simulink model "simpleprocess_controller_observer"  (Simulink 7.4)
settings: Solver=ode45  StartTime=0.0  StopTime=10.0  RelTol=1e-3
values from neighbouring files (symbols this model uses):
  Kr1 = K_ret(2)    [auslegung.m]
  Kr2 = K_ret(3)    [auslegung.m]
  Kr3 = K_ret(1)    [auslegung.m]
  Kv = 24    [auslegung.m]
undefined symbols (not defined in the file or in its folder): Kb1, Kb2, Kb3, MU1
settings Model: Creator=Alex  LastModifiedBy=Alex

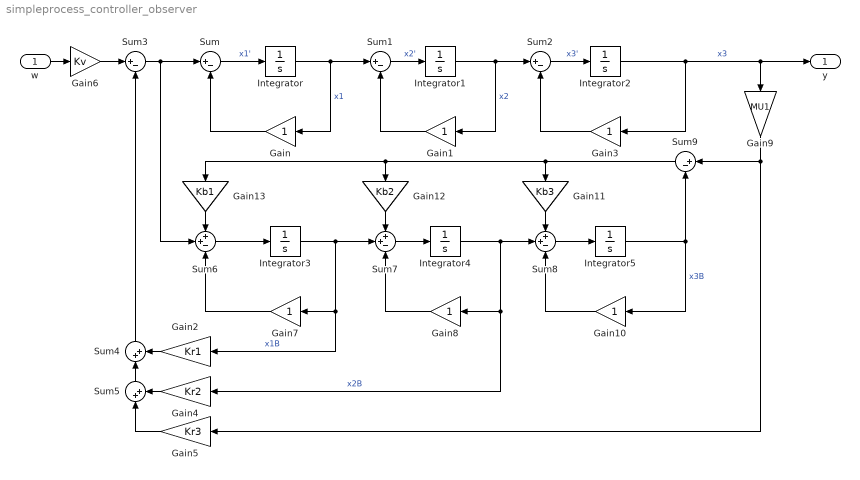
== system simpleprocess_controller_observer ==
  w : Inport  OutDataType=fixdt(1, 16)  OutScaling=2^0
  Gain{,1,3,7..8,10} (6 alike) : Gain  ParameterDataType=fixdt(1, 16)  ParameterScaling=2^0  OutDataType=fixdt(1, 16)  OutScaling=2^0
  Gain11 : Gain  Gain=Kb3  ParameterDataType=fixdt(1, 16)  ParameterScaling=2^0  OutDataType=fixdt(1, 16)  OutScaling=2^0
  Gain12 : Gain  Gain=Kb2  ParameterDataType=fixdt(1, 16)  ParameterScaling=2^0  OutDataType=fixdt(1, 16)  OutScaling=2^0
  Gain13 : Gain  Gain=Kb1  ParameterDataType=fixdt(1, 16)  ParameterScaling=2^0  OutDataType=fixdt(1, 16)  OutScaling=2^0
  Gain2 : Gain  Gain=Kr1  ParameterDataType=fixdt(1, 16)  ParameterScaling=2^0  OutDataType=fixdt(1, 16)  OutScaling=2^0
  Gain4 : Gain  Gain=Kr2  ParameterDataType=fixdt(1, 16)  ParameterScaling=2^0  OutDataType=fixdt(1, 16)  OutScaling=2^0
  Gain5 : Gain  Gain=Kr3  ParameterDataType=fixdt(1, 16)  ParameterScaling=2^0  OutDataType=fixdt(1, 16)  OutScaling=2^0
  Gain6 : Gain  Gain=Kv  ParameterDataType=fixdt(1, 16)  ParameterScaling=2^0  OutDataType=fixdt(1, 16)  OutScaling=2^0
  Gain9 : Gain  Gain=MU1  ParameterDataType=fixdt(1, 16)  ParameterScaling=2^0  OutDataType=fixdt(1, 16)  OutScaling=2^0
  Integrator{,1..5} (6 alike) : Integrator
  Sum{,1..3,9} (5 alike) : Sum  Inputs=|+-  OutDataType=fixdt(1, 16)  OutScaling=2^0
  Sum4 : Sum  Inputs=|++  OutDataType=fixdt(1, 16)  OutScaling=2^0
  Sum5 : Sum  Inputs=|++  OutDataType=fixdt(1, 16)  OutScaling=2^0
  Sum6 : Sum  Inputs=++-  OutDataType=fixdt(1, 16)  OutScaling=2^0
  Sum7 : Sum  Inputs=++-  OutDataType=fixdt(1, 16)  OutScaling=2^0
  Sum8 : Sum  Inputs=++-  OutDataType=fixdt(1, 16)  OutScaling=2^0
  y : Outport  OutDataType=fixdt(1, 16)  OutScaling=2^0
  wires:
  Gain/1 -> Sum/2
  Sum/1 -> Integrator/1  "x1'"
  Integrator2/1 -> Gain3/1, y/1, Gain9/1  "x3"
  Integrator/1 -> Sum1/1, Gain/1  "x1"
  Sum1/1 -> Integrator1/1  "x2'"
  Integrator1/1 -> Sum2/1, Gain1/1  "x2"
  Sum2/1 -> Integrator2/1  "x3'"
  Gain1/1 -> Sum1/2
  Gain3/1 -> Sum2/2
  w/1 -> Gain6/1
  Gain6/1 -> Sum3/1
  Sum3/1 -> Sum/1, Sum6/2
  Gain5/1 -> Sum5/1
  Gain4/1 -> Sum5/2
  Gain2/1 -> Sum4/2
  Sum5/1 -> Sum4/1
  Sum4/1 -> Sum3/2
  Gain9/1 -> Gain5/1, Sum9/1
  Sum6/1 -> Integrator3/1
  Integrator5/1 -> Gain10/1, Sum9/2  "x3B"
  Integrator3/1 -> Gain7/1, Gain2/1, Sum7/2  "x1B"
  Sum7/1 -> Integrator4/1
  Integrator4/1 -> Gain8/1, Gain4/1, Sum8/2  "x2B"
  Sum8/1 -> Integrator5/1
  Gain7/1 -> Sum6/3
  Sum9/1 -> Gain11/1, Gain13/1, Gain12/1
  Gain8/1 -> Sum7/3
  Gain10/1 -> Sum8/3
  Gain11/1 -> Sum8/1
  Gain12/1 -> Sum7/1
  Gain13/1 -> Sum6/1
